simulink model "chapter2_jd"  (R2016b)
settings: Solver=VariableStepAuto  StartTime=0.0  StopTime=10.0  RelTol=1e-3
PreLoadFcn:
  | load PI_output;
settings Model: Creator=training-ah  LastModifiedBy=training-ah
settings DataIOCC: ExternalInput=[PI_output_time, PI_output_data]  LoadExternalInput=on  SaveFormat=Array

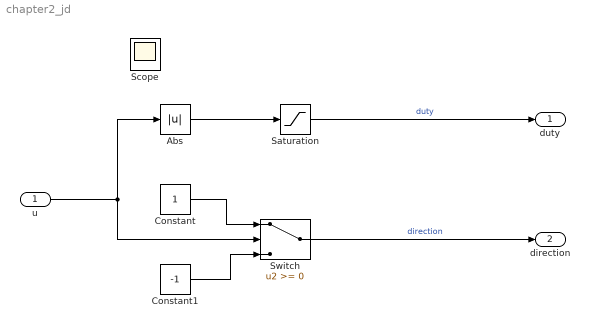
== system chapter2_jd ==
  u : Inport
  Abs : Abs
  Constant : Constant
  Constant1 : Constant  Value=-1
  Saturation : Saturate  UpperLimit=1  LowerLimit=0
  Switch : Switch
  duty : Outport
  direction : Outport  Port=2
  Scope : Scope
  wires:
  u/1 -> Switch/2, Abs/1
  Abs/1 -> Saturation/1
  Saturation/1 -> duty/1  "duty"
  Constant/1 -> Switch/1
  Constant1/1 -> Switch/3
  Switch/1 -> direction/1  "direction"
